simulink model "simulink_3_1a"  (R2025b)
settings: Solver=VariableStepAuto  StartTime=0.0  StopTime=5  RelTol=1e-3
settings Model: Creator=getrj  LastModifiedBy=owenm

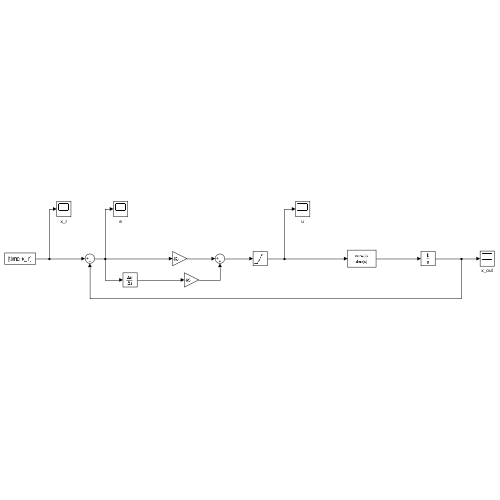
[thumbnail: Simulink's stored preview of the top-level diagram]
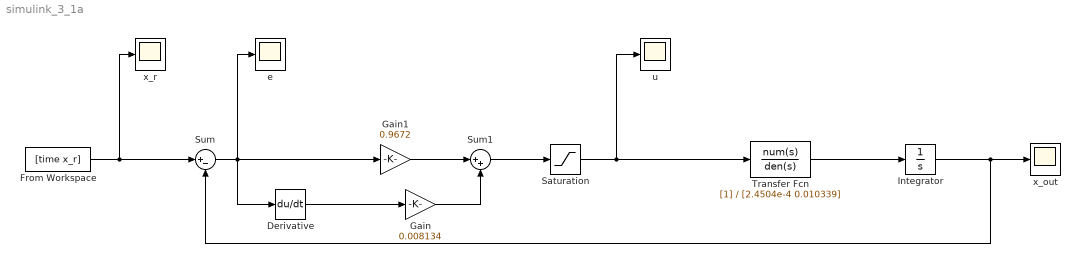
== system simulink_3_1a ==
  Derivative : Derivative
  From Workspace : FromWorkspace  VariableName=[time x_r]
  Gain : Gain  Gain=0.008134
  Gain1 : Gain  Gain=0.9672
  Integrator : Integrator
  Saturation : Saturate  UpperLimit=10  LowerLimit=-10
  Sum : Sum  Inputs=|+-
  Sum1 : Sum  Inputs=|++
  Transfer Fcn : TransferFcn  Denominator=[2.4504e-4 0.010339]
  e : Scope
      settings: ActiveDisplayYMinimum=-1.4036486042205962  ActiveDisplayYMaximum=1.4050979082872819  DataLoggingVariableName=ScopeData2
  u : Scope
      settings: ActiveDisplayYMinimum=-1.7457966026126042  ActiveDisplayYMaximum=1.792401371371751
  x_out : Scope
      settings: ActiveDisplayYMinimum=-7.7720195314384561  ActiveDisplayYMaximum=58.4293416193652
  x_r : Scope
      settings: ActiveDisplayYMinimum=-6.2499999999999982  ActiveDisplayYMaximum=56.25  DataLoggingVariableName=ScopeData3
  wires:
  From Workspace/1 -> x_r/1, Sum/1
  Sum/1 -> e/1, Derivative/1, Gain1/1
  Gain1/1 -> Sum1/1
  Gain/1 -> Sum1/2
  Sum1/1 -> Saturation/1
  Saturation/1 -> Transfer Fcn/1, u/1
  Transfer Fcn/1 -> Integrator/1
  Integrator/1 -> Sum/2, x_out/1
  Derivative/1 -> Gain/1
